simulink model "gm_test_RS_flipflop_statemachine"  (R2021a)
settings: Solver=FixedStepDiscrete  StartTime=0.0  StopTime=210*10e-8  RelTol=1e-3
undefined symbols (not defined in the file or in its folder): t_ADC, t_clock
libraries: simulink x15, hdlmdlgenlib x15, simulink_extras x4, eeGeneralControl x1
settings Model: Creator=micha  LastModifiedBy=micha
settings SolverCC: AlgebraicLoopSolver=TrustRegion
settings DataIOCC: LimitDataPoints=on  SaveOutput=off  SaveTime=off
settings OptimizationCC: BlockReduction=off  ConditionallyExecuteInputs=off  DefaultParameterBehavior=Inlined  LifeSpan=inf
settings DebuggingCC: AlgebraicLoopMsg=error  InheritedTsInSrcMsg=none  SingleTaskRateTransMsg=error  AllowSymbolicDim=off  StrictBusMsg=ErrorOnBusTreatedAsVector  SFUnexpectedBacktrackingDiag=warning  SFNoUnconditionalDefaultTransitionDiag=warning  SFExecutionAtInitializationDiag=none  SFMachineParentedDataDiag=warning  ArithmeticOperatorsInVariantConditions=warning
settings HardwareCC: ProdBitPerPointer=32  ProdBitPerSizeT=32  ProdBitPerPtrDiffT=32  ProdLargestAtomicFloat=None  ProdIntDivRoundTo=Undefined  ProdEndianess=Unspecified  ProdWordSize=32  ProdHWDeviceType=ASIC/FPGA->ASIC/FPGA  ProdEqTarget=off
settings SFSimCC: SimUseLocalCustomCode=off  CustomCodeUndefinedFunction=UseInterfaceOnly
settings RTWCC: RTWUseLocalCustomCode=off
settings CodeAppCC: StateflowObjectComments=on
settings GRTTargetCC: TargetLangStandard=C89/C90 (ANSI)
settings ConfigComp: CovScope=ReferencedModels  CovMetricSettings=dw  CovSaveCumulativeToWorkspaceVar=on  CovSaveSingleToWorkspaceVar=on  CovExternalEMLEnable=off  CovSFcnEnable=off

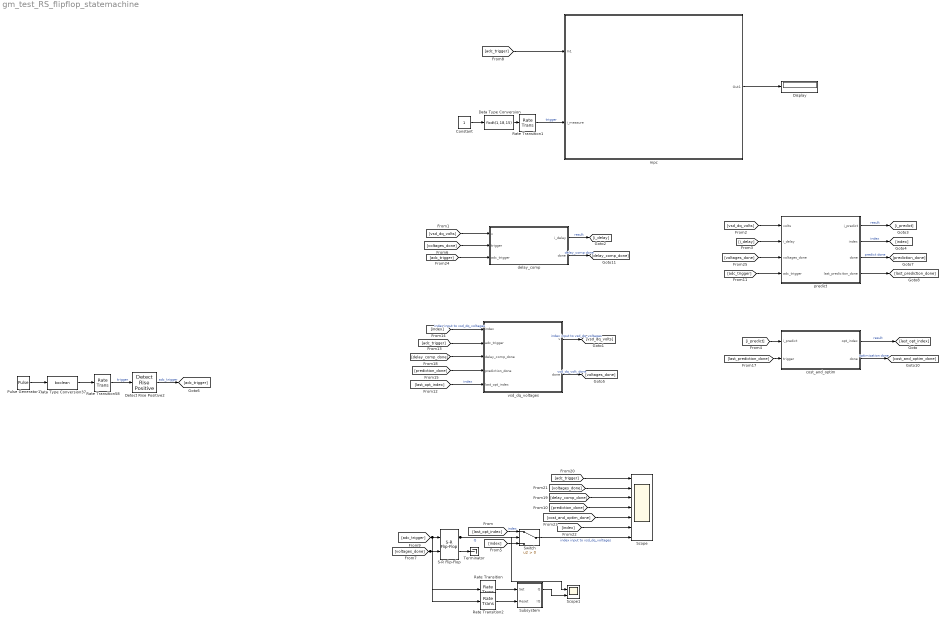
== system gm_test_RS_flipflop_statemachine ==
  Constant : Constant
  Data Type Conversion : DataTypeConversion  OutDataTypeStr=fixdt(1,18,15)
  Data Type Conversion37 : DataTypeConversion  OutDataTypeStr=boolean
  Detect Rise Positive2 : simulink/Logic and Bit Operations/Detect Rise Positive  vinit=0  OutDataTypeStr=boolean
  Display : Display
  Pulse Generator1 : DiscretePulseGenerator  PulseType=Time based  Period=t_ADC  PulseWidth=5
  Rate Transition{,1..2,58} (4 alike) : RateTransition  OutPortSampleTime=t_clock
  S-R Flip-Flop : simulink_extras/Flip Flops/S-R Flip-Flop  initial_condition=0
  Scope : Scope  NumInputPorts=7
  Scope1 : Scope  NumInputPorts=2
  Subsystem : Subsystem
  Switch : Switch  Criteria=u2 > Threshold
  Terminator : Terminator
  cost_and_optim : Subsystem
  delay_comp : Subsystem
  mpc : Subsystem  TreatAsAtomicUnit=on
  predict : Subsystem
  vsd_dq_voltages : Subsystem
  wires:
  Rate Transition2/1 -> Subsystem/2(Reset)
  Rate Transition/1 -> Subsystem/1(Set)
  Subsystem/1(Q) -> Scope1/2
  mpc/1(Out1) -> Display/1
  Data Type Conversion/1 -> Rate Transition1/1
  Constant/1 -> Data Type Conversion/1
  Rate Transition1/1 -> mpc/2(i_measure)  "trigger"
  [adc_trigger] -> mpc/1(In1)
  [prediction_done] -> Scope/4
  predict/4(last_prediciton_done) -> [last_prediction_done]
  [voltages_done] -> predict/3(voltages_done)
  delay_comp/2(done) -> [delay_comp_done]  "delay_comp done"
  [adc_trigger] -> delay_comp/3(adc_trigger)
  [cost_and_optim_done] -> Scope/5
  cost_and_optim/2(done) -> [cost_and_optim_done]  "optimization done"
  [index] -> Scope/6
  [voltages_done] -> Scope/2
  [adc_trigger] -> Scope/1
  [delay_comp_done] -> Scope/3
  Switch/1 -> Scope/7  "index input to vsd_dq_voltages"
  [delay_comp_done] -> vsd_dq_voltages/3(delay_comp_done)
  [last_prediction_done] -> cost_and_optim/2(trigger)
  [prediction_done] -> vsd_dq_voltages/4(prediction_done)
  vsd_dq_voltages/1(v) -> [vsd_dq_volts]  "index input to vsd_dq_voltages"
  [adc_trigger] -> vsd_dq_voltages/2(adc_trigger)
  [last_opt_index] -> vsd_dq_voltages/5(last_opt_index)  "index"
  [adc_trigger] -> predict/4(adc_trigger)
  [adc_trigger] -> S-R Flip-Flop/1, Rate Transition/1
  [voltages_done] -> S-R Flip-Flop/2, Rate Transition2/1
  [voltages_done] -> delay_comp/2(trigger)
  [index] -> Switch/3
  [i_predict] -> cost_and_optim/1(i_predict)
  predict/1(i_predict) -> [i_predict]  "result"
  [i_delay] -> predict/2(i_delay)
  delay_comp/1(i_delay) -> [i_delay]  "result"
  [vsd_dq_volts] -> predict/1(volts)
  [vsd_dq_volts] -> delay_comp/1(v)
  cost_and_optim/1(opt_index) -> [last_opt_index]  "result"
  predict/2(index) -> [index]  "index"
  predict/3(done) -> [prediction_done]  "predict done"
  vsd_dq_voltages/2(done) -> [voltages_done]  "vsd_dq_volt_done"
  Detect Rise Positive2/1 -> [adc_trigger]  "adc_trigger"
  S-R Flip-Flop/2 -> Terminator/1
  [index] -> vsd_dq_voltages/1(index)  "index input to vsd_dq_voltages"
  [last_opt_index] -> Switch/1  "index"
  S-R Flip-Flop/1 -> Switch/2, Scope1/1  "Q"
  Pulse Generator1/1 -> Data Type Conversion37/1
  Rate Transition58/1 -> Detect Rise Positive2/1  "trigger"
  Data Type Conversion37/1 -> Rate Transition58/1

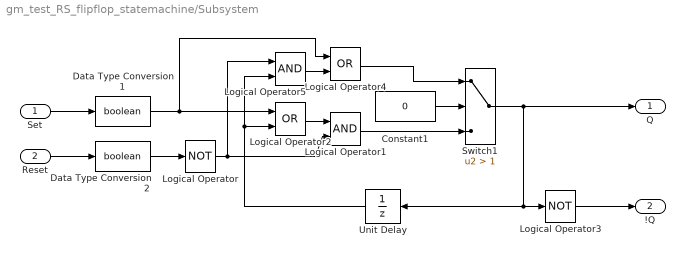
== system gm_test_RS_flipflop_statemachine/Subsystem ==
  Set : Inport
  Reset : Inport  Port=2
  Constant1 : Constant  Value=0  SampleTime=-1
  Data Type Conversion1 : DataTypeConversion  OutDataTypeStr=boolean
  Data Type Conversion2 : DataTypeConversion  OutDataTypeStr=boolean
  Logical Operator : Logic  Operator=NOT  AllPortsSameDT=off  OutDataTypeStr=boolean
  Logical Operator1 : Logic  AllPortsSameDT=off  OutDataTypeStr=boolean
  Logical Operator2 : Logic  Operator=OR  AllPortsSameDT=off  OutDataTypeStr=boolean
  Logical Operator3 : Logic  Operator=NOT  AllPortsSameDT=off  OutDataTypeStr=boolean
  Logical Operator4 : Logic  Operator=OR  AllPortsSameDT=off  OutDataTypeStr=boolean
  Logical Operator5 : Logic  AllPortsSameDT=off  OutDataTypeStr=boolean
  Switch1 : Switch  Criteria=u2 > Threshold  Threshold=1
  Unit Delay : UnitDelay  SampleTime=t_clock  HasFrameUpgradeWarning=on
  Q : Outport  VectorParamsAs1DForOutWhenUnconnected=off
  !Q : Outport  Port=2  VectorParamsAs1DForOutWhenUnconnected=off
  wires:
  Data Type Conversion2/1 -> Logical Operator/1
  Logical Operator1/1 -> Switch1/3
  Logical Operator5/1 -> Logical Operator4/2
  Unit Delay/1 -> Logical Operator5/2, Logical Operator2/2
  Logical Operator2/1 -> Logical Operator1/1
  Set/1 -> Data Type Conversion1/1
  Logical Operator3/1 -> !Q/1
  Switch1/1 -> Logical Operator3/1, Unit Delay/1, Q/1
  Data Type Conversion1/1 -> Logical Operator4/1, Logical Operator2/1
  Logical Operator4/1 -> Switch1/1
  Constant1/1 -> Switch1/2
  Reset/1 -> Data Type Conversion2/1
  Logical Operator/1 -> Logical Operator5/1, Logical Operator1/2

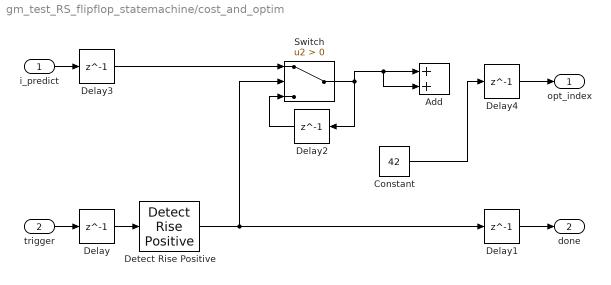
== system gm_test_RS_flipflop_statemachine/cost_and_optim ==
  i_predict : Inport
  trigger : Inport  Port=2
  Add : Sum
  Constant : Constant  Value=42
  Delay{,1..4} (5 alike) : Delay  DelayLength=1
  Detect Rise Positive : simulink/Logic and Bit Operations/Detect Rise Positive  vinit=0  OutDataTypeStr=boolean
  Switch : Switch  Criteria=u2 > Threshold
  opt_index : Outport  VectorParamsAs1DForOutWhenUnconnected=off
  done : Outport  Port=2  VectorParamsAs1DForOutWhenUnconnected=off
  wires:
  Constant/1 -> Delay4/1
  Delay4/1 -> opt_index/1
  Delay3/1 -> Switch/1
  i_predict/1 -> Delay3/1
  Switch/1 -> Delay2/1, Add/1, Add/2
  Delay2/1 -> Switch/3
  Detect Rise Positive/1 -> Switch/2, Delay1/1
  Delay1/1 -> done/1
  Delay/1 -> Detect Rise Positive/1
  trigger/1 -> Delay/1

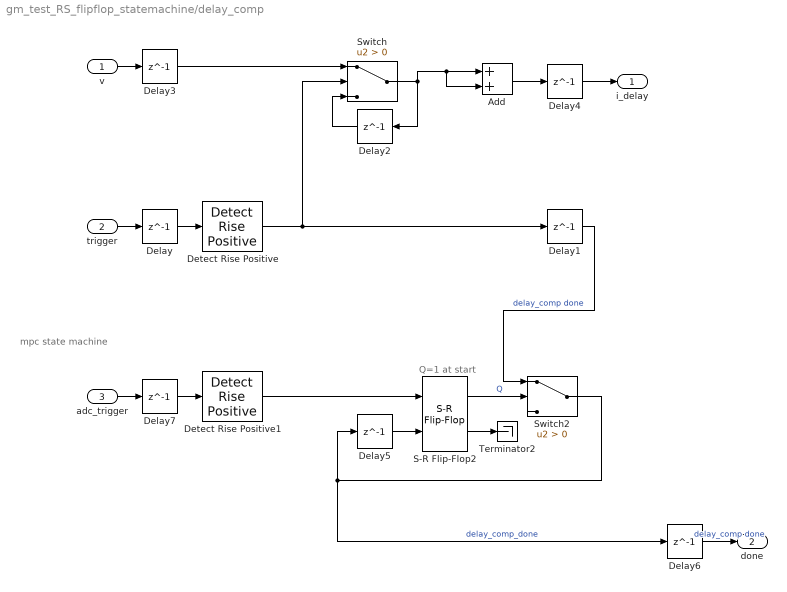
== system gm_test_RS_flipflop_statemachine/delay_comp ==
  note: Q=1 at start
  note: mpc state machine
  v : Inport
  trigger : Inport  Port=2
  adc_trigger : Inport  Port=3
  Add : Sum
  Delay{,1..7} (8 alike) : Delay  DelayLength=1
  Detect Rise Positive : simulink/Logic and Bit Operations/Detect Rise Positive  vinit=0  OutDataTypeStr=boolean
  Detect Rise Positive1 : simulink/Logic and Bit Operations/Detect Rise Positive  vinit=0  OutDataTypeStr=boolean
  S-R Flip-Flop2 : simulink_extras/Flip Flops/S-R Flip-Flop  initial_condition=1
  Switch : Switch  Criteria=u2 > Threshold
  Switch2 : Switch  Criteria=u2 > Threshold
  Terminator2 : Terminator
  i_delay : Outport  VectorParamsAs1DForOutWhenUnconnected=off
  done : Outport  Port=2  VectorParamsAs1DForOutWhenUnconnected=off
  wires:
  Detect Rise Positive1/1 -> S-R Flip-Flop2/1
  adc_trigger/1 -> Delay7/1
  Delay6/1 -> done/1  "delay_comp done"
  Delay1/1 -> Switch2/1  "delay_comp done"
  Delay5/1 -> S-R Flip-Flop2/2
  S-R Flip-Flop2/2 -> Terminator2/1
  Delay7/1 -> Detect Rise Positive1/1
  S-R Flip-Flop2/1 -> Switch2/2  "Q"
  Switch2/1 -> Delay6/1, Delay5/1  "delay_comp_done"
  Add/1 -> Delay4/1
  Delay4/1 -> i_delay/1
  Delay3/1 -> Switch/1
  v/1 -> Delay3/1
  Switch/1 -> Delay2/1, Add/1, Add/2
  Delay2/1 -> Switch/3
  Detect Rise Positive/1 -> Switch/2, Delay1/1
  Delay/1 -> Detect Rise Positive/1
  trigger/1 -> Delay/1

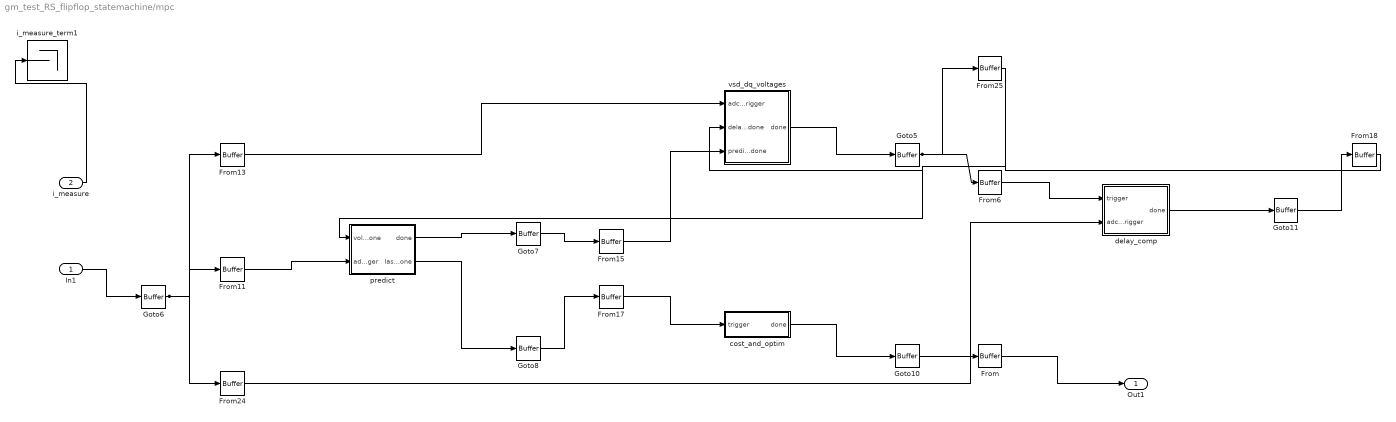
== system gm_test_RS_flipflop_statemachine/mpc ==
  In1 : Inport  OutDataTypeStr=boolean  PortDimensions=1  SampleTime=1e-08
  i_measure : Inport  Port=2  OutDataTypeStr=fixdt(1, 18, 15)  PortDimensions=1  SampleTime=1e-08
  From{,6,11,13,15,17..18,24..25} (9 alike) : hdlmdlgenlib/Buffer
      settings: SourceProductBaseCode=SL
  Goto{5..8,10..11} (6 alike) : hdlmdlgenlib/Buffer
      settings: SourceProductBaseCode=SL
  cost_and_optim : Subsystem
  delay_comp : Subsystem
  i_measure_term1 : Terminator
  predict : Subsystem
  vsd_dq_voltages : Subsystem
  Out1 : Outport  SampleTime=1e-08
  wires:
  In1/1 -> Goto6/1
  i_measure/1 -> i_measure_term1/1
  From/1 -> Out1/1
  From11/1 -> predict/2(adc_trigger)
  From13/1 -> vsd_dq_voltages/1(adc_trigger)
  From15/1 -> vsd_dq_voltages/3(prediction_done)
  From17/1 -> cost_and_optim/1(trigger)
  From18/1 -> vsd_dq_voltages/2(delay_comp_done)
  From24/1 -> delay_comp/2(adc_trigger)
  From25/1 -> predict/1(voltages_done)
  From6/1 -> delay_comp/1(trigger)
  cost_and_optim/1(done) -> Goto10/1
  delay_comp/1(done) -> Goto11/1
  predict/1(done) -> Goto7/1
  predict/2(last_prediciton_done) -> Goto8/1
  vsd_dq_voltages/1(done) -> Goto5/1
  Goto10/1 -> From/1
  Goto6/1 -> From24/1, From13/1, From11/1
  Goto7/1 -> From15/1
  Goto8/1 -> From17/1
  Goto11/1 -> From18/1
  Goto5/1 -> From6/1, From25/1

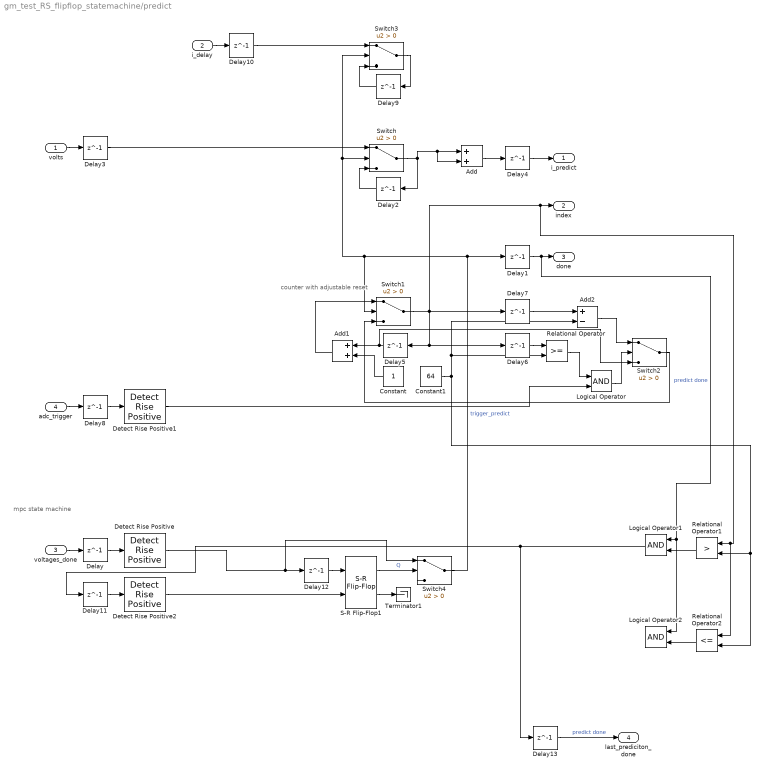
== system gm_test_RS_flipflop_statemachine/predict ==
  note: mpc state machine
  note: counter with adjustable reset
  volts : Inport
  i_delay : Inport  Port=2
  voltages_done : Inport  Port=3
  adc_trigger : Inport  Port=4
  Add : Sum
  Add1 : Sum  AccumDataTypeStr=uint32
  Add2 : Sum  Inputs=+-  AccumDataTypeStr=uint32
  Constant : Constant  OutDataTypeStr=uint32
  Constant1 : Constant  Value=64  OutDataTypeStr=uint32
  Delay{,1..4,8..13} (11 alike) : Delay  DelayLength=1
  Delay5 : Delay  DelayLength=1  InitialCondition=1
  Delay6 : Delay  DelayLength=1  InitialCondition=1
  Delay7 : Delay  DelayLength=1  InitialCondition=1
  Detect Rise Positive : simulink/Logic and Bit Operations/Detect Rise Positive  vinit=0  OutDataTypeStr=boolean
  Detect Rise Positive1 : simulink/Logic and Bit Operations/Detect Rise Positive  vinit=0  OutDataTypeStr=boolean
  Detect Rise Positive2 : simulink/Logic and Bit Operations/Detect Rise Positive  vinit=0  OutDataTypeStr=boolean
  Logical Operator : Logic  AllPortsSameDT=off  OutDataTypeStr=boolean
  Logical Operator1 : Logic  AllPortsSameDT=off  OutDataTypeStr=boolean
  Logical Operator2 : Logic  AllPortsSameDT=off  OutDataTypeStr=boolean
  Relational Operator : RelationalOperator  OutDataTypeStr=boolean  RndMeth=Simplest
  Relational Operator1 : RelationalOperator  Operator=>  OutDataTypeStr=boolean  RndMeth=Simplest
  Relational Operator2 : RelationalOperator  Operator=<=  OutDataTypeStr=boolean  RndMeth=Simplest
  S-R Flip-Flop1 : simulink_extras/Flip Flops/S-R Flip-Flop  initial_condition=0
  Switch{,1..4} (5 alike) : Switch  Criteria=u2 > Threshold
  Terminator1 : Terminator
  i_predict : Outport  VectorParamsAs1DForOutWhenUnconnected=off
  index : Outport  Port=2  VectorParamsAs1DForOutWhenUnconnected=off
  done : Outport  Port=3  VectorParamsAs1DForOutWhenUnconnected=off
  last_prediciton_done : Outport  Port=4  VectorParamsAs1DForOutWhenUnconnected=off
  wires:
  Delay13/1 -> last_prediciton_done/1  "predict done"
  Relational Operator2/1 -> Logical Operator2/2
  Delay1/1 -> done/1, Logical Operator1/1, Logical Operator2/1  "predict done"
  Switch1/1 -> index/1, Relational Operator1/1, Relational Operator2/1, Delay7/1, Delay6/1, Delay5/1
  Relational Operator1/1 -> Logical Operator1/2
  S-R Flip-Flop1/1 -> Switch4/2  "Q"
  S-R Flip-Flop1/2 -> Terminator1/1
  Delay12/1 -> S-R Flip-Flop1/1
  Detect Rise Positive/1 -> Delay12/1, Switch4/1
  Detect Rise Positive2/1 -> S-R Flip-Flop1/2
  Switch4/1 -> Switch1/2, Switch/2, Switch3/2, Delay1/1  "trigger_predict"
  Logical Operator1/1 -> Delay11/1, Delay13/1
  Delay11/1 -> Detect Rise Positive2/1
  Switch3/1 -> Delay9/1
  Delay10/1 -> Switch3/1
  Delay9/1 -> Switch3/3
  i_delay/1 -> Delay10/1
  Detect Rise Positive1/1 -> Logical Operator/2
  adc_trigger/1 -> Delay8/1
  Delay8/1 -> Detect Rise Positive1/1
  Logical Operator/1 -> Switch2/2
  Delay7/1 -> Add2/1
  Delay6/1 -> Relational Operator/1
  Add2/1 -> Switch2/1
  Switch2/1 -> Switch1/3
  Relational Operator/1 -> Logical Operator/1
  Constant1/1 -> Relational Operator/2, Add2/2, Relational Operator1/2, Relational Operator2/2
  Add1/1 -> Switch1/1
  Constant/1 -> Add1/2
  Delay5/1 -> Add1/1, Switch2/3
  Add/1 -> Delay4/1
  Delay4/1 -> i_predict/1
  Delay3/1 -> Switch/1
  volts/1 -> Delay3/1
  Switch/1 -> Delay2/1, Add/1, Add/2
  Delay2/1 -> Switch/3
  Delay/1 -> Detect Rise Positive/1
  voltages_done/1 -> Delay/1

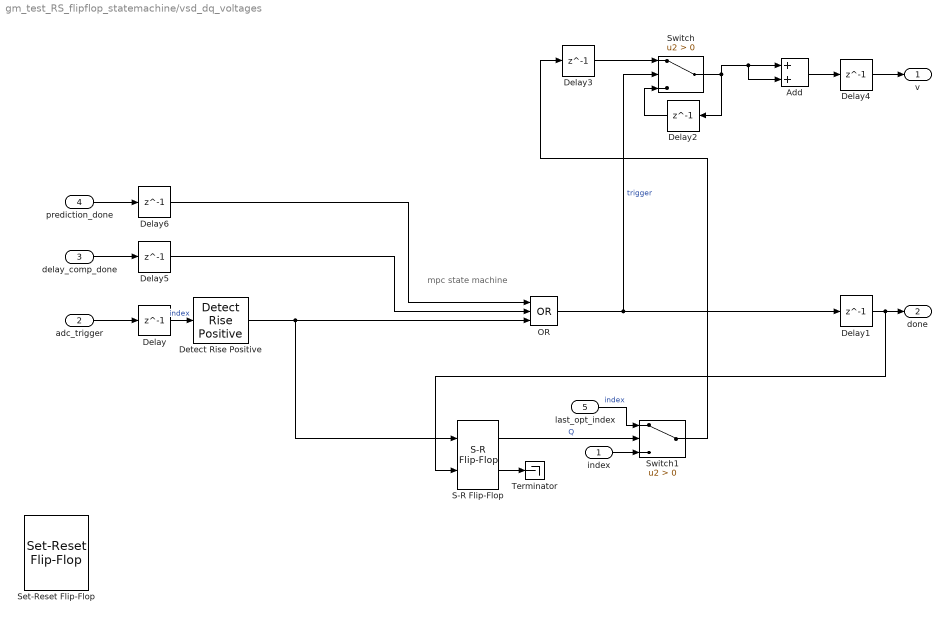
== system gm_test_RS_flipflop_statemachine/vsd_dq_voltages ==
  note: mpc state machine
  index : Inport
  adc_trigger : Inport  Port=2
  delay_comp_done : Inport  Port=3
  prediction_done : Inport  Port=4
  last_opt_index : Inport  Port=5
  Add : Sum
  Delay{,1..6} (7 alike) : Delay  DelayLength=1
  Detect Rise Positive : simulink/Logic and Bit Operations/Detect Rise Positive  vinit=0  OutDataTypeStr=boolean
  OR : Logic  Operator=OR  Inputs=3  IconShape=distinctive  AllPortsSameDT=off  OutDataTypeStr=boolean
  S-R Flip-Flop : simulink_extras/Flip Flops/S-R Flip-Flop  initial_condition=0
  Set-Reset Flip-Flop : eeGeneralControl/Set-Reset Flip-Flop  LabelModeActiveChoice=Discrete  UndefState=Set  Q0=0  Ts=-1
      settings: SourceProductBaseCode=PS
  Switch : Switch  Criteria=u2 > Threshold
  Switch1 : Switch  Criteria=u2 > Threshold
  Terminator : Terminator
  v : Outport  VectorParamsAs1DForOutWhenUnconnected=off
  done : Outport  Port=2  VectorParamsAs1DForOutWhenUnconnected=off
  wires:
  Delay/1 -> Detect Rise Positive/1  "index"
  last_opt_index/1 -> Switch1/1  "index"
  S-R Flip-Flop/1 -> Switch1/2  "Q"
  index/1 -> Switch1/3
  S-R Flip-Flop/2 -> Terminator/1
  Delay6/1 -> OR/1
  Delay5/1 -> OR/2
  prediction_done/1 -> Delay6/1
  delay_comp_done/1 -> Delay5/1
  OR/1 -> Delay1/1, Switch/2  "trigger"
  Detect Rise Positive/1 -> OR/3, S-R Flip-Flop/1
  adc_trigger/1 -> Delay/1
  Add/1 -> Delay4/1
  Delay4/1 -> v/1
  Delay3/1 -> Switch/1
  Switch1/1 -> Delay3/1
  Switch/1 -> Delay2/1, Add/1, Add/2
  Delay2/1 -> Switch/3
  Delay1/1 -> done/1, S-R Flip-Flop/2

== system gm_test_RS_flipflop_statemachine/mpc/cost_and_optim ==
  trigger : Inport  OutDataTypeStr=boolean  PortDimensions=1  SampleTime=1e-08
  Delay : Delay  DelayLength=double(1)  InitialCondition=0  SampleTime=1e-08
  Delay1 : Delay  DelayLength=double(1)  InitialCondition=0  SampleTime=1e-08
  Detect Rise Positive : simulink/Logic and Bit Operations/Detect Rise Positive  vinit=0  OutDataTypeStr=boolean
  done : Outport  SampleTime=1e-08  VectorParamsAs1DForOutWhenUnconnected=off
  wires:
  trigger/1 -> Delay/1
  Delay/1 -> Detect Rise Positive/1
  Delay1/1 -> done/1
  Detect Rise Positive/1 -> Delay1/1

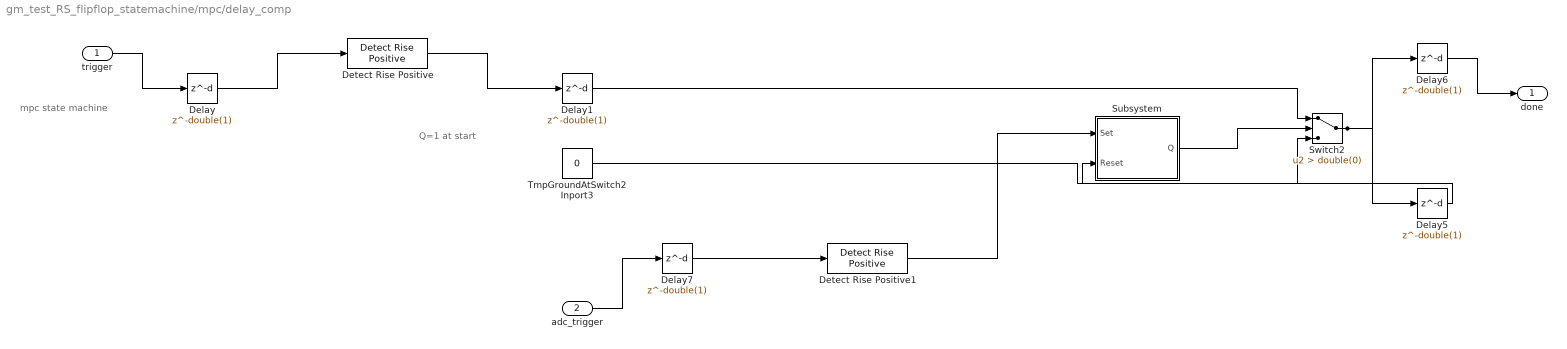
== system gm_test_RS_flipflop_statemachine/mpc/delay_comp ==
  note: Q=1 at start
  note: mpc state machine
  trigger : Inport  OutDataTypeStr=boolean  PortDimensions=1  SampleTime=1e-08
  adc_trigger : Inport  Port=2  OutDataTypeStr=boolean  PortDimensions=1  SampleTime=1e-08
  Delay{,1,5..7} (5 alike) : Delay  DelayLength=double(1)  InitialCondition=0  SampleTime=1e-08
  Detect Rise Positive : simulink/Logic and Bit Operations/Detect Rise Positive  vinit=0  OutDataTypeStr=boolean
  Detect Rise Positive1 : simulink/Logic and Bit Operations/Detect Rise Positive  vinit=0  OutDataTypeStr=boolean
  Subsystem : Subsystem
  Switch2 : Switch  Criteria=u2 > Threshold  Threshold=double(0)  OutDataTypeStr=boolean  SampleTime=1e-08
  TmpGroundAtSwitch2Inport3 : Constant  Value=0  VectorParams1D=off  OutDataTypeStr=boolean
  done : Outport  SampleTime=1e-08  VectorParamsAs1DForOutWhenUnconnected=off
  wires:
  trigger/1 -> Delay/1
  adc_trigger/1 -> Delay7/1
  Delay/1 -> Detect Rise Positive/1
  Delay1/1 -> Switch2/1
  Delay5/1 -> Subsystem/2(Reset)
  Delay6/1 -> done/1
  Delay7/1 -> Detect Rise Positive1/1
  Detect Rise Positive/1 -> Delay1/1
  Detect Rise Positive1/1 -> Subsystem/1(Set)
  Subsystem/1(Q) -> Switch2/2
  Switch2/1 -> Delay6/1, Delay5/1
  TmpGroundAtSwitch2Inport3/1 -> Switch2/3

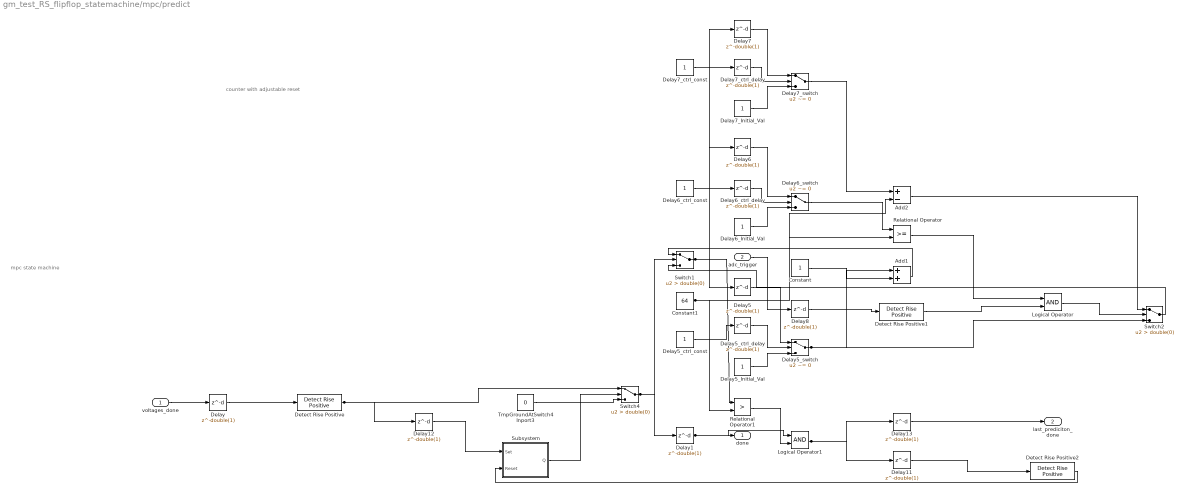
== system gm_test_RS_flipflop_statemachine/mpc/predict ==
  note: mpc state machine
  note: counter with adjustable reset
  voltages_done : Inport  OutDataTypeStr=boolean  PortDimensions=1  SampleTime=1e-08
  adc_trigger : Inport  Port=2  OutDataTypeStr=boolean  PortDimensions=1  SampleTime=1e-08
  Add1 : Sum  AccumDataTypeStr=uint32  OutDataTypeStr=uint32  SampleTime=1e-08
  Add2 : Sum  Inputs=+-  AccumDataTypeStr=uint32  OutDataTypeStr=uint32  SampleTime=1e-08
  Constant : Constant  OutDataTypeStr=uint32  SampleTime=1e-08
  Constant1 : Constant  Value=64  OutDataTypeStr=uint32  SampleTime=1e-08
  Delay{,1,5..8,11..13} (9 alike) : Delay  DelayLength=double(1)  InitialCondition=0  SampleTime=1e-08
  Delay5_Initial_Val : Constant  OutDataTypeStr=uint32  SampleTime=1e-08
  Delay5_ctrl_const : Constant  OutDataTypeStr=boolean  SampleTime=1e-08
  Delay5_ctrl_delay : Delay  DelayLength=double(1)  InitialCondition=0  SampleTime=1e-08
  Delay5_switch : Switch  Criteria=u2 ~= 0  Threshold=double(0)  OutDataTypeStr=uint32  SampleTime=1e-08
  Delay6_Initial_Val : Constant  OutDataTypeStr=uint32  SampleTime=1e-08
  Delay6_ctrl_const : Constant  OutDataTypeStr=boolean  SampleTime=1e-08
  Delay6_ctrl_delay : Delay  DelayLength=double(1)  InitialCondition=0  SampleTime=1e-08
  Delay6_switch : Switch  Criteria=u2 ~= 0  Threshold=double(0)  OutDataTypeStr=uint32  SampleTime=1e-08
  Delay7_Initial_Val : Constant  OutDataTypeStr=uint32  SampleTime=1e-08
  Delay7_ctrl_const : Constant  OutDataTypeStr=boolean  SampleTime=1e-08
  Delay7_ctrl_delay : Delay  DelayLength=double(1)  InitialCondition=0  SampleTime=1e-08
  Delay7_switch : Switch  Criteria=u2 ~= 0  Threshold=double(0)  OutDataTypeStr=uint32  SampleTime=1e-08
  Detect Rise Positive : simulink/Logic and Bit Operations/Detect Rise Positive  vinit=0  OutDataTypeStr=boolean
  Detect Rise Positive1 : simulink/Logic and Bit Operations/Detect Rise Positive  vinit=0  OutDataTypeStr=boolean
  Detect Rise Positive2 : simulink/Logic and Bit Operations/Detect Rise Positive  vinit=0  OutDataTypeStr=boolean
  Logical Operator : Logic  AllPortsSameDT=off  OutDataTypeStr=boolean  SampleTime=1e-08
  Logical Operator1 : Logic  AllPortsSameDT=off  OutDataTypeStr=boolean  SampleTime=1e-08
  Relational Operator : RelationalOperator  OutDataTypeStr=boolean  SampleTime=1e-08  RndMeth=Nearest
  Relational Operator1 : RelationalOperator  Operator=>  OutDataTypeStr=boolean  SampleTime=1e-08  RndMeth=Nearest
  Subsystem : Subsystem
  Switch1 : Switch  Criteria=u2 > Threshold  Threshold=double(0)  OutDataTypeStr=uint32  SampleTime=1e-08
  Switch2 : Switch  Criteria=u2 > Threshold  Threshold=double(0)  OutDataTypeStr=uint32  SampleTime=1e-08
  Switch4 : Switch  Criteria=u2 > Threshold  Threshold=double(0)  OutDataTypeStr=boolean  SampleTime=1e-08
  TmpGroundAtSwitch4Inport3 : Constant  Value=0  VectorParams1D=off  OutDataTypeStr=boolean
  done : Outport  SampleTime=1e-08  VectorParamsAs1DForOutWhenUnconnected=off
  last_prediciton_done : Outport  Port=2  SampleTime=1e-08  VectorParamsAs1DForOutWhenUnconnected=off
  wires:
  voltages_done/1 -> Delay/1
  adc_trigger/1 -> Delay8/1
  Add1/1 -> Switch1/1
  Add2/1 -> Switch2/1
  Constant/1 -> Add1/2
  Constant1/1 -> Relational Operator1/2, Relational Operator/2, Add2/2
  Delay/1 -> Detect Rise Positive/1
  Delay1/1 -> Logical Operator1/1, done/1
  Delay11/1 -> Detect Rise Positive2/1
  Delay12/1 -> Subsystem/1(Set)
  Delay13/1 -> last_prediciton_done/1
  Delay5_switch/1 -> Switch2/3, Add1/1
  Delay6_switch/1 -> Relational Operator/1
  Delay7_switch/1 -> Add2/1
  Delay8/1 -> Detect Rise Positive1/1
  Detect Rise Positive/1 -> Switch4/1, Delay12/1
  Detect Rise Positive1/1 -> Logical Operator/2
  Detect Rise Positive2/1 -> Subsystem/2(Reset)
  Logical Operator/1 -> Switch2/2
  Logical Operator1/1 -> Delay13/1, Delay11/1
  Relational Operator/1 -> Logical Operator/1
  Relational Operator1/1 -> Logical Operator1/2
  Subsystem/1(Q) -> Switch4/2
  Switch1/1 -> Relational Operator1/1, Delay7/1, Delay6/1, Delay5/1
  Switch2/1 -> Switch1/3
  Switch4/1 -> Switch1/2, Delay1/1
  TmpGroundAtSwitch4Inport3/1 -> Switch4/3
  Delay5/1 -> Delay5_switch/1
  Delay5_Initial_Val/1 -> Delay5_switch/3
  Delay5_ctrl_const/1 -> Delay5_ctrl_delay/1
  Delay5_ctrl_delay/1 -> Delay5_switch/2
  Delay6/1 -> Delay6_switch/1
  Delay6_Initial_Val/1 -> Delay6_switch/3
  Delay6_ctrl_const/1 -> Delay6_ctrl_delay/1
  Delay6_ctrl_delay/1 -> Delay6_switch/2
  Delay7/1 -> Delay7_switch/1
  Delay7_Initial_Val/1 -> Delay7_switch/3
  Delay7_ctrl_const/1 -> Delay7_ctrl_delay/1
  Delay7_ctrl_delay/1 -> Delay7_switch/2

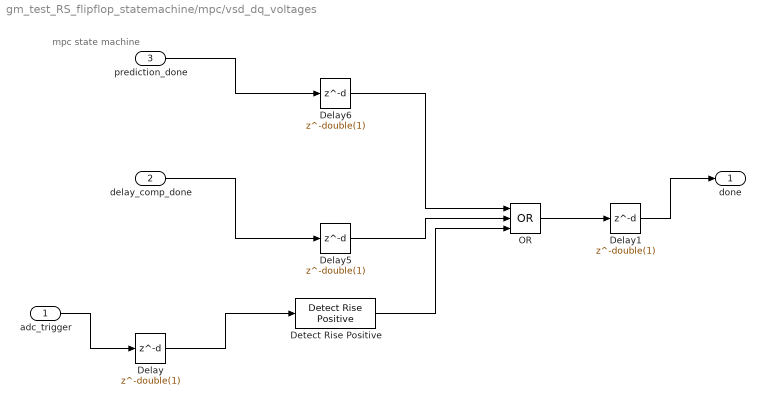
== system gm_test_RS_flipflop_statemachine/mpc/vsd_dq_voltages ==
  note: mpc state machine
  adc_trigger : Inport  OutDataTypeStr=boolean  PortDimensions=1  SampleTime=1e-08
  delay_comp_done : Inport  Port=2  OutDataTypeStr=boolean  PortDimensions=1  SampleTime=1e-08
  prediction_done : Inport  Port=3  OutDataTypeStr=boolean  PortDimensions=1  SampleTime=1e-08
  Delay{,1,5..6} (4 alike) : Delay  DelayLength=double(1)  InitialCondition=0  SampleTime=1e-08
  Detect Rise Positive : simulink/Logic and Bit Operations/Detect Rise Positive  vinit=0  OutDataTypeStr=boolean
  OR : Logic  Operator=OR  Inputs=3  AllPortsSameDT=off  OutDataTypeStr=boolean  SampleTime=1e-08
  done : Outport  SampleTime=1e-08  VectorParamsAs1DForOutWhenUnconnected=off
  wires:
  adc_trigger/1 -> Delay/1
  delay_comp_done/1 -> Delay5/1
  prediction_done/1 -> Delay6/1
  Delay/1 -> Detect Rise Positive/1
  Delay1/1 -> done/1
  Delay5/1 -> OR/2
  Delay6/1 -> OR/1
  Detect Rise Positive/1 -> OR/3
  OR/1 -> Delay1/1

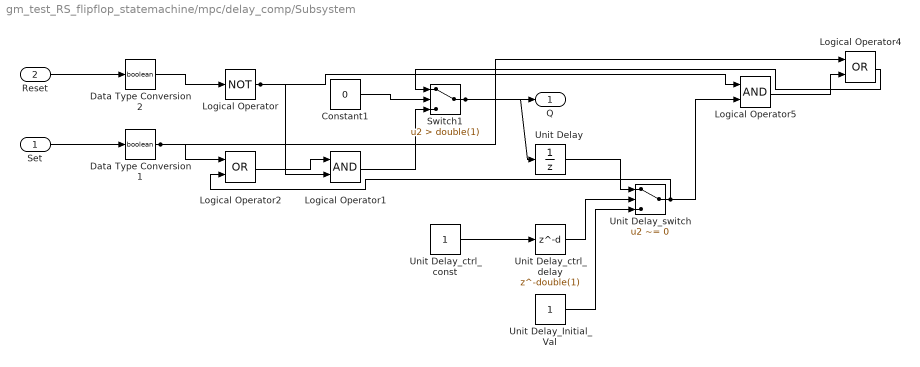
== system gm_test_RS_flipflop_statemachine/mpc/delay_comp/Subsystem ==
  Set : Inport  OutDataTypeStr=boolean  PortDimensions=1  SampleTime=1e-08
  Reset : Inport  Port=2  OutDataTypeStr=boolean  PortDimensions=1  SampleTime=1e-08
  Constant1 : Constant  Value=0  OutDataTypeStr=uint32  SampleTime=1e-08
  Data Type Conversion1 : DataTypeConversion  OutDataTypeStr=boolean  SampleTime=1e-08
  Data Type Conversion2 : DataTypeConversion  OutDataTypeStr=boolean  SampleTime=1e-08
  Logical Operator : Logic  Operator=NOT  Inputs=1  AllPortsSameDT=off  OutDataTypeStr=boolean  SampleTime=1e-08
  Logical Operator1 : Logic  AllPortsSameDT=off  OutDataTypeStr=boolean  SampleTime=1e-08
  Logical Operator2 : Logic  Operator=OR  AllPortsSameDT=off  OutDataTypeStr=boolean  SampleTime=1e-08
  Logical Operator4 : Logic  Operator=OR  AllPortsSameDT=off  OutDataTypeStr=boolean  SampleTime=1e-08
  Logical Operator5 : Logic  AllPortsSameDT=off  OutDataTypeStr=boolean  SampleTime=1e-08
  Switch1 : Switch  Criteria=u2 > Threshold  Threshold=double(1)  OutDataTypeStr=boolean  SampleTime=1e-08
  Unit Delay : UnitDelay  InitialCondition=double(0)  SampleTime=1e-08
  Unit Delay_Initial_Val : Constant  OutDataTypeStr=boolean  SampleTime=1e-08
  Unit Delay_ctrl_const : Constant  OutDataTypeStr=boolean  SampleTime=1e-08
  Unit Delay_ctrl_delay : Delay  DelayLength=double(1)  InitialCondition=0  SampleTime=1e-08
  Unit Delay_switch : Switch  Criteria=u2 ~= 0  Threshold=double(0)  OutDataTypeStr=boolean  SampleTime=1e-08
  Q : Outport  SampleTime=1e-08  VectorParamsAs1DForOutWhenUnconnected=off
  wires:
  Set/1 -> Data Type Conversion1/1
  Reset/1 -> Data Type Conversion2/1
  Constant1/1 -> Switch1/2
  Data Type Conversion1/1 -> Logical Operator4/1, Logical Operator2/1
  Data Type Conversion2/1 -> Logical Operator/1
  Logical Operator/1 -> Logical Operator5/1, Logical Operator1/2
  Logical Operator1/1 -> Switch1/3
  Logical Operator2/1 -> Logical Operator1/1
  Logical Operator4/1 -> Switch1/1
  Logical Operator5/1 -> Logical Operator4/2
  Switch1/1 -> Unit Delay/1, Q/1
  Unit Delay_switch/1 -> Logical Operator5/2, Logical Operator2/2
  Unit Delay/1 -> Unit Delay_switch/1
  Unit Delay_Initial_Val/1 -> Unit Delay_switch/3
  Unit Delay_ctrl_const/1 -> Unit Delay_ctrl_delay/1
  Unit Delay_ctrl_delay/1 -> Unit Delay_switch/2

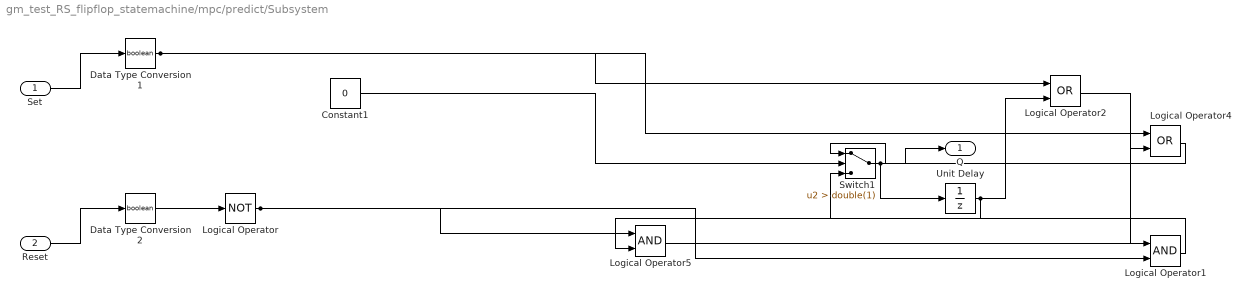
== system gm_test_RS_flipflop_statemachine/mpc/predict/Subsystem ==
  Set : Inport  OutDataTypeStr=boolean  PortDimensions=1  SampleTime=1e-08
  Reset : Inport  Port=2  OutDataTypeStr=boolean  PortDimensions=1  SampleTime=1e-08
  Constant1 : Constant  Value=0  OutDataTypeStr=uint32  SampleTime=1e-08
  Data Type Conversion1 : DataTypeConversion  OutDataTypeStr=boolean  SampleTime=1e-08
  Data Type Conversion2 : DataTypeConversion  OutDataTypeStr=boolean  SampleTime=1e-08
  Logical Operator : Logic  Operator=NOT  Inputs=1  AllPortsSameDT=off  OutDataTypeStr=boolean  SampleTime=1e-08
  Logical Operator1 : Logic  AllPortsSameDT=off  OutDataTypeStr=boolean  SampleTime=1e-08
  Logical Operator2 : Logic  Operator=OR  AllPortsSameDT=off  OutDataTypeStr=boolean  SampleTime=1e-08
  Logical Operator4 : Logic  Operator=OR  AllPortsSameDT=off  OutDataTypeStr=boolean  SampleTime=1e-08
  Logical Operator5 : Logic  AllPortsSameDT=off  OutDataTypeStr=boolean  SampleTime=1e-08
  Switch1 : Switch  Criteria=u2 > Threshold  Threshold=double(1)  OutDataTypeStr=boolean  SampleTime=1e-08
  Unit Delay : UnitDelay  SampleTime=1e-08
  Q : Outport  SampleTime=1e-08  VectorParamsAs1DForOutWhenUnconnected=off
  wires:
  Set/1 -> Data Type Conversion1/1
  Reset/1 -> Data Type Conversion2/1
  Constant1/1 -> Switch1/2
  Data Type Conversion1/1 -> Logical Operator4/1, Logical Operator2/1
  Data Type Conversion2/1 -> Logical Operator/1
  Logical Operator/1 -> Logical Operator5/1, Logical Operator1/2
  Logical Operator1/1 -> Switch1/3
  Logical Operator2/1 -> Logical Operator1/1
  Logical Operator4/1 -> Switch1/1
  Logical Operator5/1 -> Logical Operator4/2
  Switch1/1 -> Unit Delay/1, Q/1
  Unit Delay/1 -> Logical Operator5/2, Logical Operator2/2
